simulink model "shifter_start1"  (R2018b)
settings: Solver=FixedStepAuto  StartTime=0.0  StopTime=30  FixedStep=0.05  RelTol=1e-3  EnableMultiTasking=on
undefined symbols (not defined in the file): up_threshold, vehicle_speed
settings Model: Creator=jrivitus  LastModifiedBy=Alexander
settings DataIOCC: ExternalInput=[t, up_threshold, vehicle_speed, down_threshold]  LimitDataPoints=on  LoadExternalInput=on  SaveFormat=Array
settings OptimizationCC: ExpressionDepthLimit=2147483647  LifeSpan=inf
settings DebuggingCC: UnderspecifiedInitializationDetection=Classic  MergeDetectMultiDrivingBlocksExec=none  ParameterPrecisionLossMsg=none  FcnCallInpInsideContextMsg=warning  AllowSymbolicDim=off  StateNameClashWarn=warning  LibraryContextMissingDiagnostic=none  SFUnexpectedBacktrackingDiag=warning  SFNoUnconditionalDefaultTransitionDiag=warning  SFExecutionAtInitializationDiag=none
settings HardwareCC: ProdBitPerPointer=32  ProdBitPerSizeT=32  ProdBitPerPtrDiffT=32  ProdLargestAtomicFloat=None  ProdIntDivRoundTo=Undefined  ProdEndianess=Unspecified  ProdWordSize=32  ProdHWDeviceType=32-bit Generic
settings ModelReferenceCC: PropagateSignalLabelsOutOfModel=off
settings SFSimCC: SimUseLocalCustomCode=off
settings RTWCC: RTWUseLocalCustomCode=off
settings CodeAppCC: StateflowObjectComments=on
settings GRTTargetCC: TargetLangStandard=C89/C90 (ANSI)  GeneratePreprocessorConditionals=Disable all  CombineOutputUpdateFcns=off  GRTInterface=on
settings ConfigComp: CovMetricSettings=dw  CovHtmlReporting=on  CovSaveCumulativeToWorkspaceVar=on  CovSaveSingleToWorkspaceVar=on  CovExternalEMLEnable=off  CovSFcnEnable=off

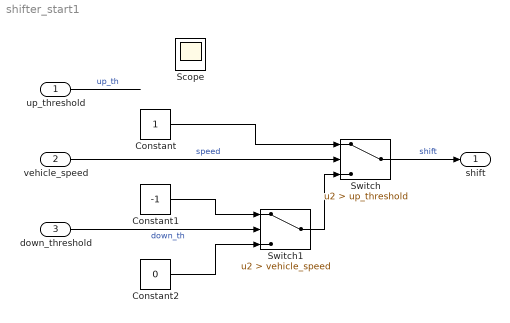
== system shifter_start1 ==
  up_threshold : Inport  OutDataTypeStr=double
  vehicle_speed : Inport  Port=2  OutDataTypeStr=double
  down_threshold : Inport  Port=3  OutDataTypeStr=double
  Constant : Constant
  Constant1 : Constant  Value=-1
  Constant2 : Constant  Value=0
  Switch : Switch  Criteria=u2 > Threshold  Threshold=up_threshold
  Switch1 : Switch  Criteria=u2 > Threshold  Threshold=vehicle_speed
  shift : Outport
  Scope : Scope
  wires:
  up_threshold/1 -> ?  "up_th"
  vehicle_speed/1 -> Switch/2  "speed"
  down_threshold/1 -> Switch1/2  "down_th"
  Switch/1 -> shift/1  "shift"
  Constant1/1 -> Switch1/1
  Constant2/1 -> Switch1/3
  Constant/1 -> Switch/1
  Switch1/1 -> Switch/3
